simulink model "UR3_Kinematics"  (R2017a)
settings: Solver=VariableStepAuto  StartTime=0.0  StopTime=inf  RelTol=1e-3  EnableMultiTasking=on
libraries: vrlib x7, simulink x6, UR3_Lib x3, dspsigattribs x1
settings Model: Creator=jorgemartins  LastModifiedBy=dscat
settings DataIOCC: LimitDataPoints=on
settings OptimizationCC: LifeSpan=inf
settings DebuggingCC: AllowSymbolicDim=off  SFUnexpectedBacktrackingDiag=warning  SFNoUnconditionalDefaultTransitionDiag=warning  SFExecutionAtInitializationDiag=none
settings ModelReferenceCC: PropagateSignalLabelsOutOfModel=off
settings GRTTargetCC: TargetLangStandard=C89/C90 (ANSI)
settings ConfigComp: CovMetricSettings=dw  CovHtmlReporting=on  CovSaveCumulativeToWorkspaceVar=on  CovSaveSingleToWorkspaceVar=on  CovExternalEMLEnable=off

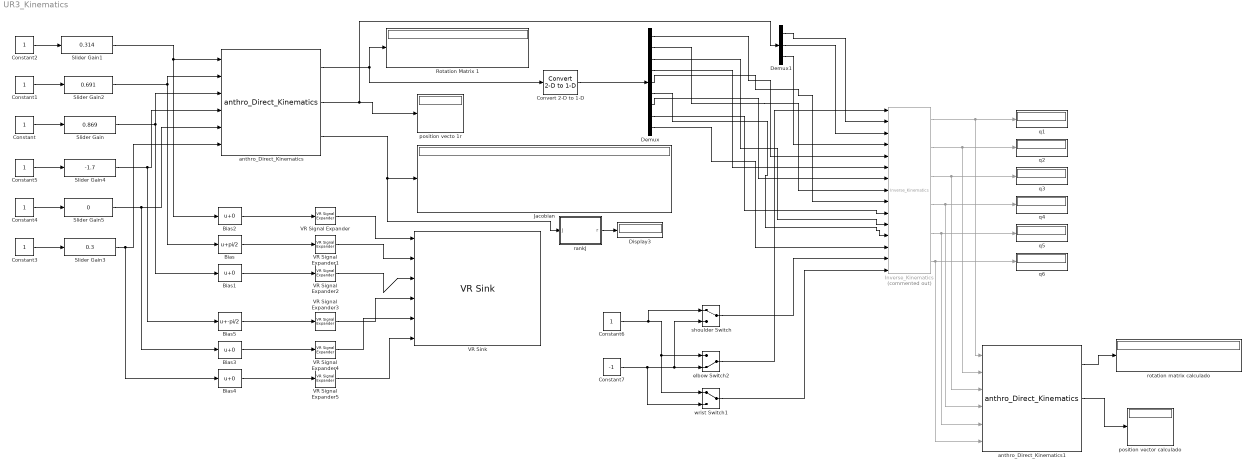
== system UR3_Kinematics ==
  Bias : Bias  Bias=pi/2
  Bias{1..4} (4 alike) : Bias
  Bias5 : Bias  Bias=-pi/2
  Constant{,1..6} (7 alike) : Constant
  Constant7 : Constant  Value=-1
  Convert 2-D to 1-D : dspsigattribs/Convert 2-D to 1-D
      settings: SourceProductName=DSP System Toolbox  SourceProductBaseCode=DS
  Demux : Demux  Outputs=9
  Demux1 : Demux  Outputs=3
  Display3 : Display
  Inverse_Kinematics : UR3_Lib/Inverse_Kinematics  Commented=on
  Jacobian : Display
  Rotation Matrix 1 : Display
  Slider Gain : simulink/Math Operations/Slider Gain  gain=0.869  low=-3.14  high=3.14
  Slider Gain1 : simulink/Math Operations/Slider Gain  gain=0.314  low=-3.14  high=3.14
  Slider Gain2 : simulink/Math Operations/Slider Gain  gain=0.691  low=-3.14  high=3.14
  Slider Gain3 : simulink/Math Operations/Slider Gain  gain=0.3  low=-1  high=1
  Slider Gain4 : simulink/Math Operations/Slider Gain  gain=-1.7  low=-3.14  high=3.14
  Slider Gain5 : simulink/Math Operations/Slider Gain  gain=0  low=-3.14  high=3.14
  VR Signal Expander{,1..5} (6 alike) : vrlib/VR Signal Expander  outwidth=4  outidx=[4]
      settings: SourceProductName=Simulink 3D Animation  SourceProductBaseCode=VR
  VR Sink : vrlib/VR Sink  InstantiateOnLoad=on  SampleTime=-1  ViewEnable=on  RemoteChange=off  RemoteView=off  FieldsWritten=Jt1_DH_dv.rotation.4.1.1.double#Jt2_DH_dv.rotation.4.1.1.double#Jt3_DH_dv.rotation.4.1.1.double#Jt4_DH_dv.rotation.4.1.1.double#Jt5_DH_dv.rotation.4.1.1.double#Jt6_DH_dv.rotation.4.1.1.double  WorldFileName=vrrobot.wrl  WorldDescription=D-H Reference Frames for Virtual Reality Robot  AutoView=on  VideoDimensions=[]  AllowVariableSize=off
      settings: SourceProductBaseCode=VR
  anthro_Direct_Kinematics : UR3_Lib/anthro_Direct_Kinematics
  anthro_Direct_Kinematics1 : UR3_Lib/anthro_Direct_Kinematics
  elbow Switch2 : ManualSwitch  CurrentSetting=0
  position vecto 1r : Display
  position vector calculado : Display
  q{1..6} (6 alike) : Display
      q1 settings: Decimation=2
  rankJ : MATLAB Function  TreatAsAtomicUnit=on
  rotation matrix calculado : Display
  shoulder Switch : ManualSwitch
  wrist Switch1 : ManualSwitch
  wires:
  anthro_Direct_Kinematics/2 -> Demux1/1, position vecto 1r/1
  Constant/1 -> Slider Gain/1
  Slider Gain/1 -> anthro_Direct_Kinematics/3, Bias1/1
  Constant2/1 -> Slider Gain1/1
  Slider Gain1/1 -> anthro_Direct_Kinematics/1, Bias2/1
  Constant1/1 -> Slider Gain2/1
  Slider Gain2/1 -> anthro_Direct_Kinematics/2, Bias/1
  Bias/1 -> VR Signal Expander1/1
  Bias1/1 -> VR Signal Expander2/1
  Bias2/1 -> VR Signal Expander/1
  Constant4/1 -> Slider Gain5/1
  Constant3/1 -> Slider Gain3/1
  Constant5/1 -> Slider Gain4/1
  Slider Gain4/1 -> anthro_Direct_Kinematics/4, Bias5/1
  Slider Gain5/1 -> anthro_Direct_Kinematics/5, Bias3/1
  Slider Gain3/1 -> anthro_Direct_Kinematics/6, Bias4/1
  Bias5/1 -> VR Signal Expander3/1
  Bias3/1 -> VR Signal Expander4/1
  Bias4/1 -> VR Signal Expander5/1
  VR Signal Expander/1 -> VR Sink/1
  VR Signal Expander1/1 -> VR Sink/2
  VR Signal Expander2/1 -> VR Sink/3
  VR Signal Expander3/1 -> VR Sink/4
  VR Signal Expander4/1 -> VR Sink/5
  VR Signal Expander5/1 -> VR Sink/6
  anthro_Direct_Kinematics/3 -> Jacobian/1, rankJ/1(J)
  rankJ/1(r) -> Display3/1
  Inverse_Kinematics/6 -> anthro_Direct_Kinematics1/6, q6/1
  Convert 2-D to 1-D/1 -> Demux/1
  Demux/1 -> Inverse_Kinematics/5
  Demux/2 -> Inverse_Kinematics/8
  Demux/3 -> Inverse_Kinematics/11
  Demux/4 -> Inverse_Kinematics/6
  Demux/5 -> Inverse_Kinematics/9
  Demux/6 -> Inverse_Kinematics/12
  Demux/7 -> Inverse_Kinematics/7
  Demux/8 -> Inverse_Kinematics/10
  Demux/9 -> Inverse_Kinematics/13
  Demux1/1 -> Inverse_Kinematics/2
  Demux1/2 -> Inverse_Kinematics/3
  Demux1/3 -> Inverse_Kinematics/4
  Inverse_Kinematics/1 -> anthro_Direct_Kinematics1/1, q1/1
  Inverse_Kinematics/2 -> anthro_Direct_Kinematics1/2, q2/1
  Inverse_Kinematics/3 -> anthro_Direct_Kinematics1/3, q3/1
  Inverse_Kinematics/4 -> anthro_Direct_Kinematics1/4, q4/1
  Inverse_Kinematics/5 -> anthro_Direct_Kinematics1/5, q5/1
  anthro_Direct_Kinematics/1 -> Rotation Matrix 1/1, Convert 2-D to 1-D/1
  Constant7/1 -> elbow Switch2/2, shoulder Switch/2, wrist Switch1/2
  Constant6/1 -> elbow Switch2/1, wrist Switch1/1, shoulder Switch/1
  shoulder Switch/1 -> Inverse_Kinematics/14
  elbow Switch2/1 -> Inverse_Kinematics/1
  wrist Switch1/1 -> Inverse_Kinematics/15
  anthro_Direct_Kinematics1/1 -> rotation matrix calculado/1
  anthro_Direct_Kinematics1/2 -> position vector calculado/1

== matlab function UR3_Kinematics/rankJ ==
  data: J input; r output
function r = rankJ(J)

r = rank(J);
end
